simulink model "binaryBaseband"  (R2020b)
settings: Solver=VariableStepAuto  StartTime=0.0  StopTime=8*Tb  RelTol=1e-3
undefined symbols (not defined in the file): A, initial_seed, Ns, Tb, Ts
libraries: commfilt2 x1, commrandsrc3 x1
settings Model: Creator=Leo Duran  LastModifiedBy=Leo Duran

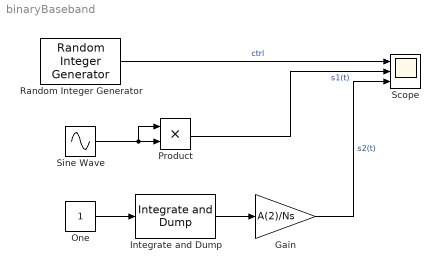
== system binaryBaseband ==
  Gain : Gain  Gain=A(2)/Ns
  Integrate and Dump : commfilt2/Integrate and Dump  obssamples=Ns  offsetsamples=0  nodump=on  roundingMode=Floor  overflowMode=off  outputDataTypeStr=Inherit: Same as accumulator  outputLastDataTypeStr=Inherit: Same as accumulator
  One : Constant  OutDataTypeStr=Inherit: Inherit via back propagation
  Product : Product
  Random Integer Generator : commrandsrc3/Random Integer Generator  SetSize=2  SeedSource=Parameter  Seed=initial_seed  SampleTime=Tb  SamplesPerFrame=1  OutputDataType=double  SimulateUsing=Interpreted execution
  Scope : Scope  NumInputPorts=3
  Sine Wave : Sin  SineType=Sample based  Amplitude=sqrt(A(1))  Samples=2*Ns  SampleTime=Ts
  wires:
  Random Integer Generator/1 -> Scope/1  "ctrl"
  Sine Wave/1 -> Product/1, Product/2
  Product/1 -> Scope/2  "s1(t)"
  One/1 -> Integrate and Dump/1
  Integrate and Dump/1 -> Gain/1
  Gain/1 -> Scope/3  "s2(t)"
